simulink model "AngleModel"  (R2021b)
settings: Solver=VariableStepAuto  StartTime=0.0  StopTime=1  RelTol=1e-3
values from neighbouring files (symbols this model uses):
  J = 0.0023    [Lab1.m]
  Mst = J*Wnls/Tm    [Lab1.m]
  Wnls = x(1)    [Lab1.m]    (also in code_by_myself.m = final_array_of_Wnls_Tm(1))
settings Model: Creator=romas  LastModifiedBy=huynh

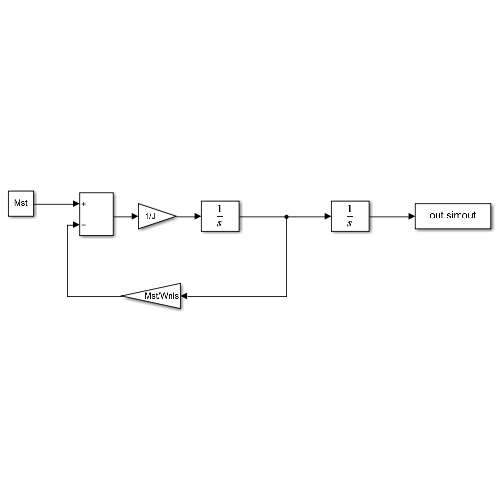
[thumbnail: Simulink's stored preview of the top-level diagram]
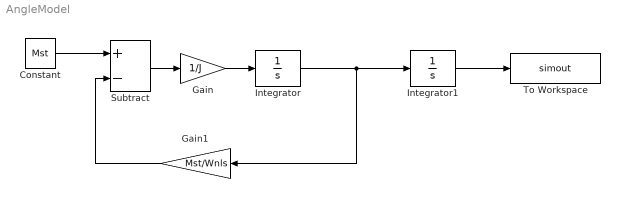
== system AngleModel ==
  Constant : Constant  Value=Mst
  Gain : Gain  Gain=1/J
  Gain1 : Gain  Gain=Mst/Wnls
  Integrator : Integrator
  Integrator1 : Integrator
  Subtract : Sum  Inputs=+-
  To Workspace : ToWorkspace  VariableName=simout  SaveFormat=Timeseries  SampleTime=-1
  wires:
  Constant/1 -> Subtract/1
  Gain1/1 -> Subtract/2
  Subtract/1 -> Gain/1
  Gain/1 -> Integrator/1
  Integrator/1 -> Integrator1/1, Gain1/1
  Integrator1/1 -> To Workspace/1
